simulink model "simulink_21uec072"  (R2022b)
settings: Solver=VariableStepAuto  StartTime=0.0  StopTime=0.0  RelTol=1e-3
settings Model: Creator=DSP-27  LastModifiedBy=DSP-27

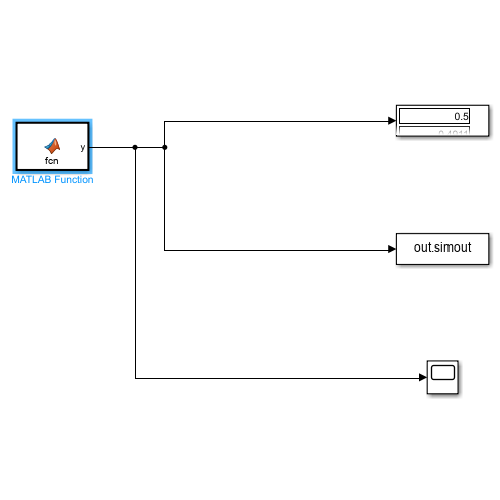
[thumbnail: Simulink's stored preview of the top-level diagram]
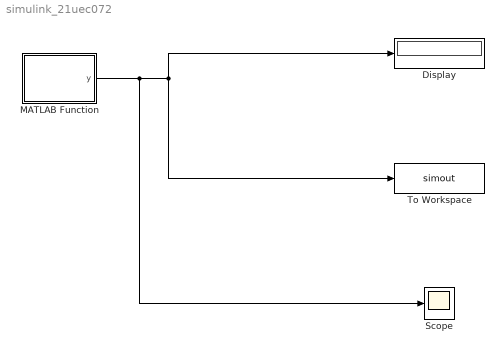
== system simulink_21uec072 ==
  Display : Display
  MATLAB Function : MATLAB Function  TreatAsAtomicUnit=on
  Scope : Scope
  To Workspace : ToWorkspace  VariableName=simout  SampleTime=-1
      settings: Save2DSignal=2-D array (concatenate along first dimension)
  wires:
  MATLAB Function/1(y) -> Scope/1, To Workspace/1, Display/1

== matlab function simulink_21uec072/MATLAB Function ==
  data: y output
function y = fcn()

Fs=1e5;
f=3e3;
n=0:1:ceil(5*Fs/f);
A=0.5;
Xs = A.*cos(2*pi*f*n*(1/Fs));
y = Xs';
